simulink model "cruisecontrol"  (R2021b)
settings: Solver=VariableStepAuto  StartTime=0.0  StopTime=t  RelTol=1e-3
values from neighbouring files (symbols this model uses):
  k = 0.5*rho*A*Cd/m    [longitudinal.m]
  kd = 470    [longitudinal.m]
  ki = 850    [longitudinal.m]
  kp = 2000    [longitudinal.m]
  m = M(i)    [longitudinal.m]
  r = 3    [longitudinal.m]
  ts = 20    [longitudinal.m]
  x = 0.5*m*k^0.5    [longitudinal.m]
settings Model: Creator=Dikshita Kothari  LastModifiedBy=Dikshita Kothari

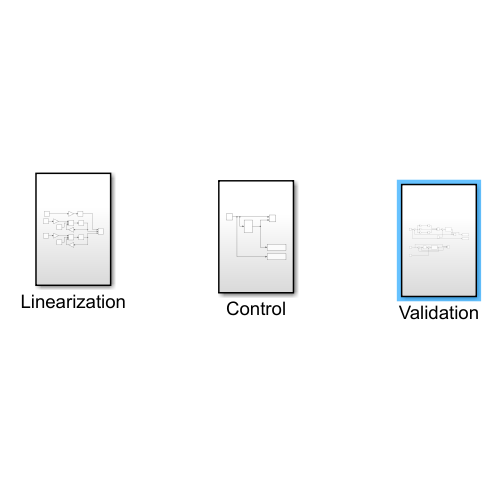
[thumbnail: Simulink's stored preview of the top-level diagram]
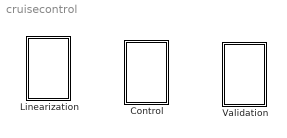
== system cruisecontrol ==
  Control : Subsystem
  Linearization : Subsystem
  Validation : Subsystem

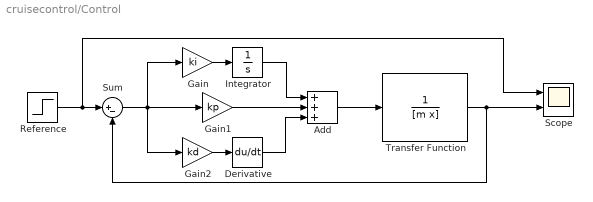
== system cruisecontrol/Control ==
  Add : Sum  Inputs=+++
  Derivative : Derivative
  Gain : Gain  Gain=ki
  Gain1 : Gain  Gain=kp
  Gain2 : Gain  Gain=kd
  Integrator : Integrator
  Reference : Step  Time=0  After=r  SampleTime=0
  Scope : Scope  NumInputPorts=2
  Sum : Sum  Inputs=|+-
  Transfer Function : TransferFcn  Denominator=[m x]
  wires:
  Transfer Function/1 -> Sum/2, Scope/2
  Add/1 -> Transfer Function/1
  Derivative/1 -> Add/3
  Gain2/1 -> Derivative/1
  Gain1/1 -> Add/2
  Integrator/1 -> Add/1
  Gain/1 -> Integrator/1
  Sum/1 -> Gain/1, Gain2/1, Gain1/1
  Reference/1 -> Sum/1, Scope/1

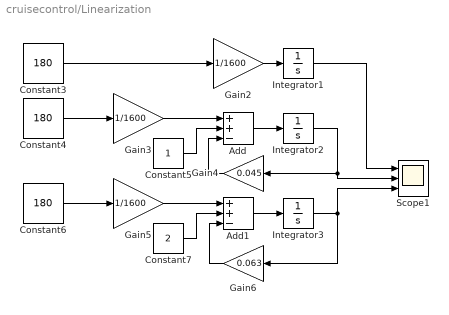
== system cruisecontrol/Linearization ==
  Add : Sum  Inputs=++-
  Add1 : Sum  Inputs=++-
  Constant3 : Constant  Value=180
  Constant4 : Constant  Value=180
  Constant5 : Constant
  Constant6 : Constant  Value=180
  Constant7 : Constant  Value=2
  Gain2 : Gain  Gain=1/1600
  Gain3 : Gain  Gain=1/1600
  Gain4 : Gain  Gain=0.045
  Gain5 : Gain  Gain=1/1600
  Gain6 : Gain  Gain=0.063
  Integrator1 : Integrator
  Integrator2 : Integrator
  Integrator3 : Integrator
  Scope1 : Scope  NumInputPorts=3
  wires:
  Integrator2/1 -> Gain4/1, Scope1/2
  Constant6/1 -> Gain5/1
  Integrator1/1 -> Scope1/1
  Gain6/1 -> Add1/3
  Integrator3/1 -> Gain6/1, Scope1/3
  Constant4/1 -> Gain3/1
  Constant7/1 -> Add1/2
  Gain5/1 -> Add1/1
  Add1/1 -> Integrator3/1
  Gain4/1 -> Add/3
  Constant3/1 -> Gain2/1
  Gain2/1 -> Integrator1/1
  Constant5/1 -> Add/2
  Add/1 -> Integrator2/1
  Gain3/1 -> Add/1

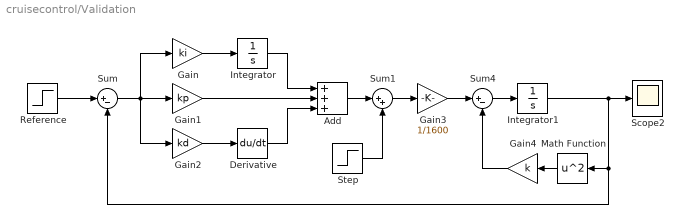
== system cruisecontrol/Validation ==
  Add : Sum  Inputs=+++
  Derivative : Derivative
  Gain : Gain  Gain=ki
  Gain1 : Gain  Gain=kp
  Gain2 : Gain  Gain=kd
  Gain3 : Gain  Gain=1/1600
  Gain4 : Gain  Gain=k
  Integrator : Integrator
  Integrator1 : Integrator
  Math Function : Math  Operator=square  SaturateOnIntegerOverflow=on
  Reference : Step  Time=0  After=r  SampleTime=0
  Scope2 : Scope
  Step : Step  Time=ts  After=-2328.144  SampleTime=0
  Sum : Sum  Inputs=|+-
  Sum1 : Sum  Inputs=|++
  Sum4 : Sum  Inputs=|+-
  wires:
  Step/1 -> Sum1/2
  Reference/1 -> Sum/1
  Gain/1 -> Integrator/1
  Integrator/1 -> Add/1
  Gain1/1 -> Add/2
  Gain2/1 -> Derivative/1
  Derivative/1 -> Add/3
  Sum/1 -> Gain2/1, Gain/1, Gain1/1
  Add/1 -> Sum1/1
  Sum1/1 -> Gain3/1
  Gain3/1 -> Sum4/1
  Gain4/1 -> Sum4/2
  Math Function/1 -> Gain4/1
  Sum4/1 -> Integrator1/1
  Integrator1/1 -> Scope2/1, Sum/2, Math Function/1
